simulink model "prystupalab8trans_si"  (R2023b)
settings: Solver=VariableStepAuto  StartTime=0.0  StopTime=10.0  RelTol=1e-3
values from neighbouring files (symbols this model uses):
  dfw1 = 0.1*fwmax1    [prystupalab8.m]
  dfw2 = 0    [prystupalab8.m]
  H01 = (fw1)/a1+H02    [prystupalab8.m]
  H02 = (fw1+fw2)/a2    [prystupalab8.m]
  L1 = [A2 a1+a2]    [prystupalab8.m]
  L2 = [a1]    [prystupalab8.m]
  L3 = [A1 a1]    [prystupalab8.m]
  L4 = [a1]    [prystupalab8.m]
  MS = [A1*A2 (A1*a1+A1*a2+A2*a1) a1*a2]    [prystupalab8.m]
  t0 = 10    [prystupalab8.m]
settings Model: Creator=Adam  LastModifiedBy=Adam

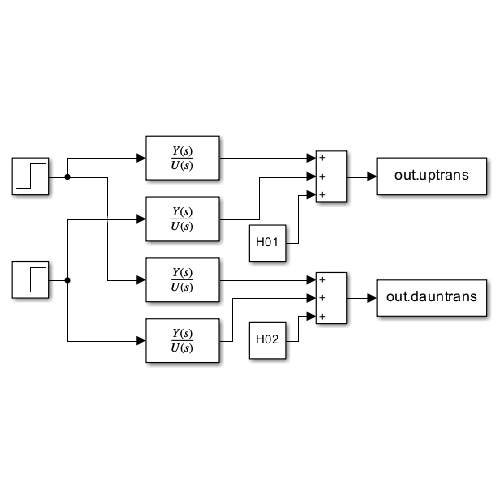
[thumbnail: Simulink's stored preview of the top-level diagram]
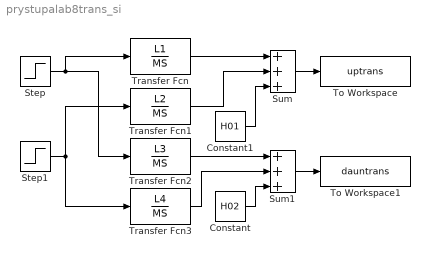
== system prystupalab8trans_si ==
  Constant : Constant  Value=H02
  Constant1 : Constant  Value=H01
  Step : Step  Time=t0  After=dfw1  SampleTime=0
  Step1 : Step  Time=t0  After=dfw2  SampleTime=0
  Sum : Sum  Inputs=+++
  Sum1 : Sum  Inputs=+++
  To Workspace : ToWorkspace  VariableName=uptrans  SampleTime=-1
  To Workspace1 : ToWorkspace  VariableName=dauntrans  SampleTime=-1
  Transfer Fcn : TransferFcn  Numerator=L1  Denominator=MS
  Transfer Fcn1 : TransferFcn  Numerator=L2  Denominator=MS
  Transfer Fcn2 : TransferFcn  Numerator=L3  Denominator=MS
  Transfer Fcn3 : TransferFcn  Numerator=L4  Denominator=MS
  wires:
  Step/1 -> Transfer Fcn2/1, Transfer Fcn/1
  Step1/1 -> Transfer Fcn3/1, Transfer Fcn1/1
  Sum1/1 -> To Workspace1/1
  Sum/1 -> To Workspace/1
  Transfer Fcn/1 -> Sum/1
  Transfer Fcn1/1 -> Sum/2
  Transfer Fcn2/1 -> Sum1/1
  Transfer Fcn3/1 -> Sum1/2
  Constant/1 -> Sum1/3
  Constant1/1 -> Sum/3
